simulink model "jasstyr"  (Simulink 10.3)
settings: Solver=ode45  StartTime=0.0  StopTime=15  RelTol=1e-3  EnableMultiTasking=on
undefined symbols (not defined in the file or in its folder): pos
libraries: cstblocks x4, simulink x1
settings Model: Creator=ola  LastModifiedBy=emiwi425  ExtModeAutoUpdateStatusClock=off
settings SolverCC: AlgebraicLoopSolver=Auto
settings DataIOCC: LimitDataPoints=on
settings OptimizationCC: ExpressionDepthLimit=128  InitFltsAndDblsToZero=on
settings DebuggingCC: SaveWithParameterizedLinksMsg=none  SignalResolutionControl=TryResolveAllWithWarning  SolverPrmCheckMsg=warning  MultiTaskDSMMsg=warning  MultiTaskCondExecSysMsg=none  StateNameClashWarn=none
settings SFSimCC: SimUseLocalCustomCode=on  CustomCodeUndefinedFunction=FilterOut
settings RTWCC: RTWUseLocalCustomCode=on
settings GRTTargetCC: TargetFcnLib=ansi_tfl_tmw.mat
settings ConfigComp: CovExternalEMLEnable=on

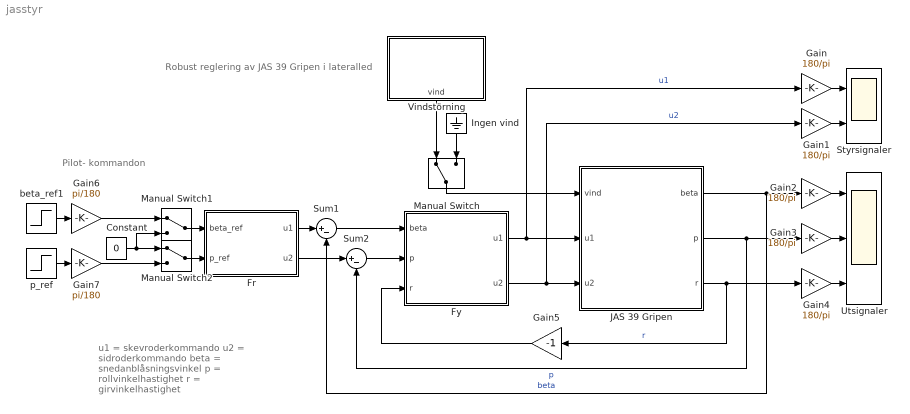
== system jasstyr ==
  note: Robust reglering av JAS 39 Gripen i lateralled
  note: Pilot-
      |  kommandon
  note: u1 = skevroderkommando
      |  u2 = sidroderkommando
      |
      |  beta = snedanblåsningsvinkel
      |  p = rollvinkelhastighet
      |  r = girvinkelhastighet
  " Ingen vind" : Ground
  " Vindstörning" : Subsystem
      mask Display: image(imread('windblow.jpg'))
  Constant : Constant  Value=0
  Fr : Subsystem
  Fy : Subsystem
  Gain{,1..4} (5 alike) : Gain  Gain=180/pi
  Gain5 : Gain  Gain=-1
  Gain6 : Gain  Gain=pi/180
  Gain7 : Gain  Gain=pi/180
  JAS 39 Gripen : Subsystem
      mask Display: image(imread('gripen.jpg'));
  Manual Switch : ManualSwitch
  Manual Switch1 : ManualSwitch
  Manual Switch2 : ManualSwitch
  Styrsignaler : Scope  NumInputPorts=2
  Sum1 : Sum  Inputs=|+-
  Sum2 : Sum  Inputs=|+-
  Utsignaler : Scope  NumInputPorts=3
  beta_ref1 : Step  Time=5  Before=5  After=0  SampleTime=0
  p_ref : Step  Time=3  Before=150  After=0  SampleTime=0
  wires:
  JAS 39 Gripen/1(beta) -> Gain2/1, Sum1/2  "beta"
  JAS 39 Gripen/2(p) -> Gain3/1, Sum2/2  "p"
  JAS 39 Gripen/3(r) -> Gain4/1, Gain5/1  "r"
  Fr/1(u1) -> Sum1/1
  Manual Switch/1 -> JAS 39 Gripen/1(vind)
  " Ingen vind"/1 -> Manual Switch/2
  " Vindstörning"/1(vind) -> Manual Switch/1
  Gain/1 -> Styrsignaler/1
  Gain1/1 -> Styrsignaler/2
  Gain2/1 -> Utsignaler/1
  Gain3/1 -> Utsignaler/2
  Gain4/1 -> Utsignaler/3
  Manual Switch1/1 -> Fr/1(beta_ref)
  Manual Switch2/1 -> Fr/2(p_ref)
  beta_ref1/1 -> Gain6/1
  p_ref/1 -> Gain7/1
  Fr/2(u2) -> Sum2/1
  Fy/1(u1) -> Gain/1, JAS 39 Gripen/2(u1)  "u1"
  Fy/2(u2) -> Gain1/1, JAS 39 Gripen/3(u2)  "u2"
  Sum1/1 -> Fy/1(beta)
  Sum2/1 -> Fy/2(p)
  Gain5/1 -> Fy/3(r)
  Constant/1 -> Manual Switch2/1, Manual Switch1/2
  Gain6/1 -> Manual Switch1/1
  Gain7/1 -> Manual Switch2/2

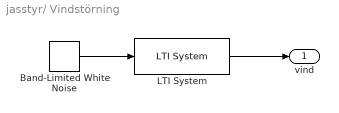
== system jasstyr/ Vindstörning ==
  Band-Limited White Noise : simulink/Sources/Band-Limited White Noise  Cov=[1 1]  Ts=0.01  seed=[23341 23342]
  LTI System : cstblocks/LTI System  sys=H  IC=0
  vind : Outport
  wires:
  LTI System/1 -> vind/1
  Band-Limited White Noise/1 -> LTI System/1

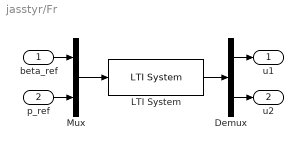
== system jasstyr/Fr ==
  beta_ref : Inport
  p_ref : Inport  Port=2
  Demux : Demux  Outputs=2
  LTI System : cstblocks/LTI System  sys=Fr  IC=[]
  Mux : Mux  Inputs=2
  u1 : Outport
  u2 : Outport  Port=2
  wires:
  beta_ref/1 -> Mux/1
  Mux/1 -> LTI System/1
  LTI System/1 -> Demux/1
  Demux/1 -> u1/1
  p_ref/1 -> Mux/2
  Demux/2 -> u2/1

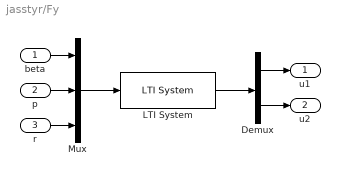
== system jasstyr/Fy ==
  beta : Inport
  p : Inport  Port=2
  r : Inport  Port=3
  Demux : Demux  Outputs=2
  LTI System : cstblocks/LTI System  sys=Fy  IC=0
  Mux : Mux  Inputs=3
  u1 : Outport
  u2 : Outport  Port=2
  wires:
  LTI System/1 -> Demux/1
  Demux/2 -> u2/1
  Demux/1 -> u1/1
  beta/1 -> Mux/1
  p/1 -> Mux/2
  r/1 -> Mux/3
  Mux/1 -> LTI System/1

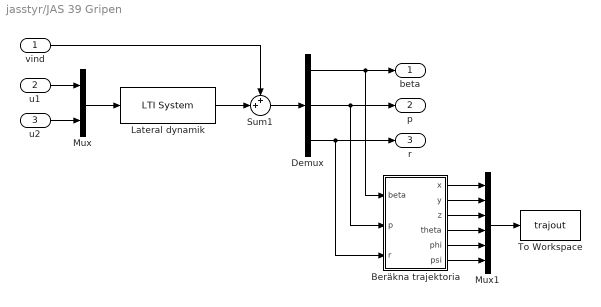
== system jasstyr/JAS 39 Gripen ==
  vind : Inport
  u1 : Inport  Port=2
  u2 : Inport  Port=3
  Beräkna trajektoria : Subsystem
  Demux : Demux  Outputs=3
  Lateral dynamik : cstblocks/LTI System  sys=G  IC=0
  Mux : Mux  Inputs=2
  Mux1 : Mux  Inputs=6
  Sum1 : Sum  Inputs=++|
  To Workspace : ToWorkspace  VariableName=trajout  SaveFormat=Structure With Time  SampleTime=.1
  beta : Outport
  p : Outport  Port=2
  r : Outport  Port=3
  wires:
  u1/1 -> Mux/1
  u2/1 -> Mux/2
  Mux/1 -> Lateral dynamik/1
  Demux/3 -> r/1, Beräkna trajektoria/3(r)
  Demux/2 -> p/1, Beräkna trajektoria/2(p)
  Demux/1 -> beta/1, Beräkna trajektoria/1(beta)
  vind/1 -> Sum1/1
  Lateral dynamik/1 -> Sum1/2
  Sum1/1 -> Demux/1
  Beräkna trajektoria/1(x) -> Mux1/1
  Beräkna trajektoria/2(y) -> Mux1/2
  Beräkna trajektoria/3(z) -> Mux1/3
  Beräkna trajektoria/4(theta) -> Mux1/4
  Beräkna trajektoria/5(phi) -> Mux1/5
  Beräkna trajektoria/6(psi) -> Mux1/6
  Mux1/1 -> To Workspace/1

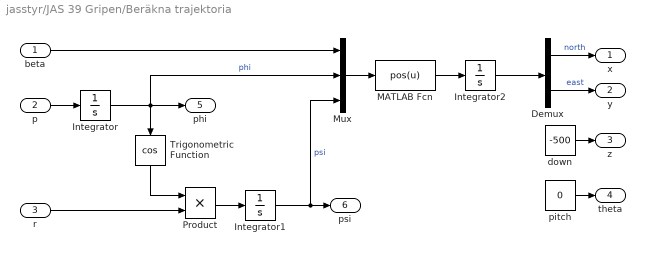
== system jasstyr/JAS 39 Gripen/Beräkna trajektoria ==
  beta : Inport
  p : Inport  Port=2
  r : Inport  Port=3
  Demux : Demux  Outputs=2
  Integrator : Integrator
  Integrator1 : Integrator
  Integrator2 : Integrator
  MATLAB Fcn : MATLABFcn  MATLABFcn=pos(u)
  Mux : Mux  Inputs=3
  Product : Product  RndMeth=Zero
  Trigonometric Function : Trigonometry  Operator=cos
  down : Constant  Value=-500
  pitch : Constant  Value=0
  x : Outport
  y : Outport  Port=2
  z : Outport  Port=3
  theta : Outport  Port=4
  phi : Outport  Port=5
  psi : Outport  Port=6
  wires:
  Demux/1 -> x/1  "north"
  Demux/2 -> y/1  "east"
  Integrator2/1 -> Demux/1
  MATLAB Fcn/1 -> Integrator2/1
  beta/1 -> Mux/1
  Mux/1 -> MATLAB Fcn/1
  Integrator1/1 -> Mux/3, psi/1  "psi"
  Product/1 -> Integrator1/1
  r/1 -> Product/2
  Trigonometric Function/1 -> Product/1
  Integrator/1 -> Mux/2, phi/1, Trigonometric Function/1  "phi"
  p/1 -> Integrator/1
  down/1 -> z/1
  pitch/1 -> theta/1
